simulink model "Nonlinear"  (R2019b)
settings: Solver=ode113  StartTime=0.0  StopTime=100  RelTol=1e-5
values from neighbouring files (symbols this model uses):
  ap = 1    [Main_Nonlinear.m]
  Gam = 2*diag([1 1 1 1 1 1])    [Main_Nonlinear.m]
  kp = 3    [Main_Nonlinear.m]
  signkp = sign(kp)    [Main_Nonlinear.m]
  theta = [0;0;0;0;0;0]    [Main_Nonlinear.m]
  theta_f = [0.01;-1;1;0.5]    [Main_Nonlinear.m]
libraries: cstblocks x1
settings Model: Creator=Thilo  LastModifiedBy=Thilo

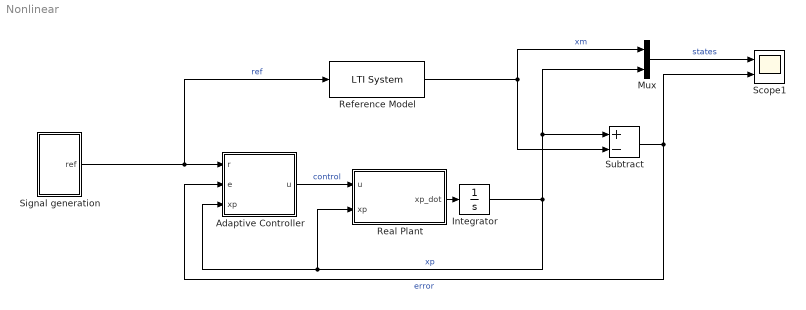
== system Nonlinear ==
  Adaptive Controller : Subsystem
  Integrator : Integrator
  Mux : Mux  Inputs=2
  Real Plant : MATLAB Function  TreatAsAtomicUnit=on
  Reference Model : cstblocks/LTI System  sys=M  IC=[0]
  Scope1 : Scope  NumInputPorts=2
  Signal generation : Subsystem
  Subtract : Sum  Inputs=+-
  wires:
  Integrator/1 -> Subtract/1, Mux/2, Adaptive Controller/3(xp), Real Plant/2(xp)  "xp"
  Adaptive Controller/1(u) -> Real Plant/1(u)  "control"
  Subtract/1 -> Scope1/2, Adaptive Controller/2(e)  "error"
  Reference Model/1 -> Subtract/2, Mux/1  "xm"
  Mux/1 -> Scope1/1  "states"
  Real Plant/1(xp_dot) -> Integrator/1
  Signal generation/1(ref) -> Reference Model/1, Adaptive Controller/1(r)  "ref"

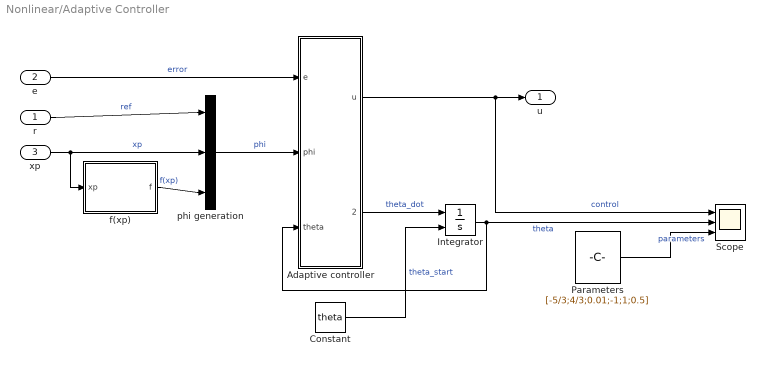
== system Nonlinear/Adaptive Controller ==
  r : Inport
  e : Inport  Port=2
  xp : Inport  Port=3
  Adaptive controller : MATLAB Function  TreatAsAtomicUnit=on
  Constant : Constant  Value=theta
  Integrator : Integrator  InitialConditionSource=external  InitialCondition=[0;0;0]
  Parameters : Constant  Value=[-5/3;4/3;0.01;-1;1;0.5]
  Scope : Scope  NumInputPorts=3
  "f(xp) " : MATLAB Function  TreatAsAtomicUnit=on
  phi generation : Concatenate  NumInputs=3
  u : Outport
  wires:
  r/1 -> phi generation/1  "ref"
  xp/1 -> "f(xp) "/1(xp), phi generation/2  "xp"
  Integrator/1 -> Scope/2, Adaptive controller/3(theta)  "theta"
  e/1 -> Adaptive controller/1(e)  "error"
  Adaptive controller/1(u) -> Scope/1, u/1  "control"
  Constant/1 -> Integrator/2  "theta_start"
  Adaptive controller/2(thetad) -> Integrator/1  "theta_dot"
  Parameters/1 -> Scope/3  "parameters"
  "f(xp) "/1(f) -> phi generation/3  "f(xp)"
  phi generation/1 -> Adaptive controller/2(phi)  "phi"

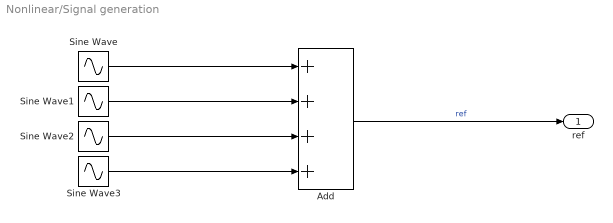
== system Nonlinear/Signal generation ==
  Add : Sum  Inputs=++++
  Sine Wave : Sin  Frequency=3  SampleTime=0
  Sine Wave1 : Sin  Frequency=3/2  SampleTime=0
  Sine Wave2 : Sin  Frequency=3/4  SampleTime=0
  Sine Wave3 : Sin  Frequency=3/8  SampleTime=0
  ref : Outport
  wires:
  Sine Wave/1 -> Add/1
  Sine Wave2/1 -> Add/3
  Sine Wave1/1 -> Add/2
  Sine Wave3/1 -> Add/4
  Add/1 -> ref/1  "ref"

== matlab function Nonlinear/Adaptive Controller/Adaptive controller ==
  data: e input; phi input; u output size=1; theta input; thetad output size=6; signkp parameter; Gam parameter
function [u,thetad] = fcn(e,phi,theta,signkp,Gam)
% Control
u = theta'*phi;
% Adpative Law
thetad = -Gam* signkp* e* phi;
% thetad = 0;

== matlab function Nonlinear/Adaptive Controller/f(xp)  ==
  data: xp input; f output; theta_f parameter
function f = fcn(xp,theta_f)
psi_f = [xp^3;exp(-10*(xp+0.5)^2);exp(-10*(xp-0.5)^2);sin(2*xp)];
f = psi_f;

== matlab function Nonlinear/Real Plant ==
  data: u input; xp_dot output; xp input; kp parameter; ap parameter; theta_f parameter
function xp_dot = fcn(u,xp,kp,ap,theta_f)
psi_f = [xp^3;exp(-10*(xp+0.5)^2);exp(-10*(xp-0.5)^2);sin(2*xp)];
xp_dot = ap*xp+kp*u-kp*theta_f'*psi_f;
